simulink model "Csm_HighLvlArchitecture"  (R2017b)
settings: Solver=VariableStepAuto  StartTime=0.0  StopTime=10.0  RelTol=1e-3
undefined symbols (not defined in the file): accEgoVeh, Acceleration, apsEgoVeh, bpEgoVeh, Coasting, Control, CurrentDrivingLane, Curvature, CutIn, CutOut, Decelleration, distEgo2TS, distPredVeh, EgoVeh_State, EgoVehicle, GRG, Idle, ITS, Localization, Management, MATLAB, Mobileye, Obstacles, Obstacles_State, Perception, posEgoVeh, posGear, posTrafficSignal, PrecedingVehicle, Prediction, Python, Regen, Run, Slope, spdEgoVeh, spdMot, spdPredVeh, SpeedLimit, SRG, Stop, Topography, Topography_State, trqMot, Type, user_define_author, user_define_category, user_define_platform, Visual_C, yawEgoVeh
libraries: DX_Lib x1
(part 1 of 2)
settings Model: Creator=Haksu  LastModifiedBy=Haksu

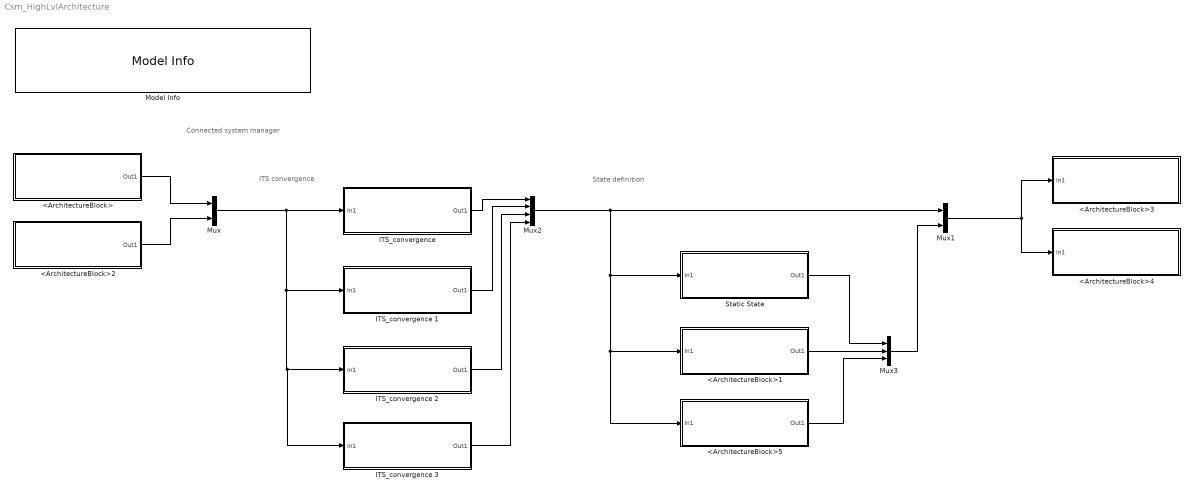
== system Csm_HighLvlArchitecture ==
  note: State definition
  note: ITS convergence
  note: Connected system manager
  <ArchitectureBlock> : Subsystem  mask{AlgorithmFullName=Localization, pop_author=__UserDef, editvalue_a=user_define_author, pop_platform=Visual_C, editvalue_p=user_define_platform, pop_category=__UserDef, editvalue_c=user_define_category, author_val=SRG, platform_val=Visual_C, algorithm_val=ITS}
      mask prompts: pop_author "Author"; editvalue_a "UserDefine"; pop_platform "Platform"; editvalue_p "UserDefine"; pop_category "Category"; editvalue_c "UserDefine"; author_val "Buff_author"; platform_val "Buff_Platform"; algorithm_val "Buff_Category"
      mask TypeOptions pop_author: Kyunghan | Haksu | Kyuhwan | Gyubin | Seungeon | __UserDef
      mask Callback pop_author:
      | % Get the mask parameter values. This is a cell
      | %   array of character vectors.
      | authorStr = get_param(gcb,'pop_author');
      | % The pop-up menu is the first mask parameter.
      | %   Check the value selected in the pop-up
      | if strcmp(authorStr(1),'_'),
      |     % Set the visibility of both parameters on when
      |     %   User-defined is selected in the pop-up.
      |     set_param(gcb,'editvalue_a','user_define_author');
      |     set_param(gcb,'MaskVisibilities',{'on';'on';'on';'on';'off';'on';'off';'off';'off';'off'}),
      |     % Get all Tab Names returned in cell array
      | 
      |     % Get visibility of all parameters
      | %     editvalStr = get_param(gcb,'editvalue')
      | %     set_param(gcb,'author_val',editvalStr)
      | else
      | 
      |     % Turn off the visibility of the Value field
      |     %   when User-defined is not selected.
      | 
      |     set_param(gcb,'MaskVisibilities',{'on';'on';'off';'on';'off';'on';'off';'off';'off';'off'}),
      |     % Set the character vector in the Values field equal to the
      |     % character vector selected in the Gain pop-up menu.
      | 
      |     %maskStr{2}=maskStr{1};
      | %     set_param(gcb,'author_val',authorStr);
      | end
      mask TypeOptions pop_platform: MATLAB | Python | Visual_C | __UserDef
      mask Callback pop_platform:
      | % Get the mask parameter values. This is a cell
      | %   array of character vectors.
      | platformSet = get_param(gcb,'pop_platform');
      | % The pop-up menu is the first mask parameter.
      | %   Check the value selected in the pop-up
      | if strcmp(platformSet(1),'_'),
      |     % Set the visibility of both parameters on when
      |     %   User-defined is selected in the pop-up.
      |     set_param(gcb,'editvalue_p','user_define_platform')
      |     set_param(gcb,'MaskVisibilities',{'on';'on';'off';'on';'on';'on';'off';'off';'off';'off'}),
      |     % Get all Tab Names returned in cell array
      | 
      |     % Get visibility of all parameters
      | %     editvalStr = get_param(gcb,'editvalue')
      | %     set_param(gcb,'platform_val',editvalStr)
      | else
      | 
      |     % Turn off the visibility of the Value field
      |     %   when User-defined is not selected.
      | 
      |     set_param(gcb,'MaskVisibilities',{'on';'on';'off';'on';'off';'on';'off';'off';'off';'off'}),
      |     % Set the character vector in the Values field equal to the
      |     % character vector selected in the Gain pop-up menu.
      | 
      |     %maskStr{2}=maskStr{1};
      | %     set_param(gcb,'platform_val',platformSet);
      | end
      mask TypeOptions pop_category: Management | Prediction | Control | __UserDef
      mask Callback pop_category:
      | % Get the mask parameter values. This is a cell
      | %   array of character vectors.
      | categoryset = get_param(gcb,'pop_category');
      | % The pop-up menu is the first mask parameter.
      | %   Check the value selected in the pop-up
      | if strcmp(categoryset(1),'_'),
      |     % Set the visibility of both parameters on when
      |     %   User-defined is selected in the pop-up.
      |     set_param(gcb,'editvalue_c','user_define_category')
      |     set_param(gcb,'MaskVisibilities',{'on';'on';'off';'on';'off';'on';'on';'off';'off';'off'}),
      |     % Get all Tab Names returned in cell array
      | else
      |     % Turn off the visibility of the Value field
      |     %   when User-defined is not selected.
      |     set_param(gcb,'MaskVisibilities',{'on';'on';'off';'on';'off';'on';'off';'off';'off';'off'}),
      |     % Set the character vector in the Values field equal to the
      |     % character vector selected in the Gain pop-up menu.
      |     %maskStr{2}=maskStr{1};
      | end
      mask DialogControl DescGroupVar Prompt: Description
      mask DialogControl DescTextVar Prompt: %<AlgorithmFullName>
      mask DialogControl ParamDesc Prompt: Description
      mask DialogControl Text1 Prompt: Author: %<author_val>
      mask DialogControl Text2 Prompt: Platform: %<platform_val>
      mask DialogControl Text3 Prompt: Algorithm: %<algorithm_val>
      mask DialogControl ParameterGroupVar Prompt: SetParam
      mask DialogControl Control5 Prompt: Set
      mask DialogControl Control5 Callback:
      | authorset = get_param(gcb,'pop_author');
      | platformset = get_param(gcb,'pop_platform');
      | categoryset = get_param(gcb,'pop_category');
      | % The pop-up menu is the first mask parameter.
      | %   Check the value selected in the pop-up
      | if strcmp(authorset(1),'_'),
      |     editvalStr = get_param(gcb,'editvalue_a');
      |     set_param(gcb,'author_val',editvalStr);
      | else
      |     set_param(gcb,'author_val',authorset);
      | end
      | 
      | if strcmp(platformset(1),'_'),
      |     editvalStr = get_param(gcb,'editvalue_p');
      |     set_param(gcb,'platform_val',editvalStr);
      | else
      |     set_param(gcb,'platform_val',platformset);
      | end
      | 
      | if strcmp(categoryset(1),'_'),
      |     editvalStr = get_param(gcb,'editvalue_c');
      |     set_param(gcb,'algorithm_val',editvalStr);
      | else
      |     set_param(gcb,'algorithm_val',categoryset);
      | end
      mask Display:
      | val_dis_author = get_param(gcb,'author_val');
      | val_dis_plat = get_param(gcb,'platform_val');
      | val_dis_cat = get_param(gcb,'algorithm_val');
      | val_dis_desc = get_param(gcb,'AlgorithmFullName');
      | 
      | colorstr = 'black';
      | switch(val_dis_cat)
      |     case 'Management'
      |         colorstr = 'lightblue';
      |     case 'Prediction'
      |         colorstr = 'blue';
      |     case 'Control'
      |         colorstr = 'green';
      |     otherwise
      |         colorstr = 'yellow';
      | end
      | 
      | % if val_dis_cat == 'Management'
      | %     colorstr = 'lightblue';
      | % end
      | % if val_dis_cat == 'Prediction'
      | %     colorstr = 'blue';
      | % end
      | 
      | % if val_dis_cat == 'Control'
      | %     colorstr = 'blue';
      | % end
      | % if val_dis_cat == 'Control'
      | %     colorstr = 'green';
      | % end
      | 
      | color(colorstr);
      | text(0.5,0.9,val_dis_desc,'horizontalAlignment', 'center', 'VerticalAlignment','Top');
      | color('black');
      | fprintf('\nAuthor: %s\nPlatform: %s\nCategory: %s',val_dis_author,val_dis_plat,val_dis_cat);
  <ArchitectureBlock>1 : Subsystem  mask{AlgorithmFullName=Obstacles_State, pop_author=__UserDef, editvalue_a=user_define_author, pop_platform=Python, editvalue_p=user_define_platform, pop_category=Management, editvalue_c=user_define_category, author_val=user_define_author, platform_val=Python, algorithm_val=Management}
      mask prompts: pop_author "Author"; editvalue_a "UserDefine"; pop_platform "Platform"; editvalue_p "UserDefine"; pop_category "Category"; editvalue_c "UserDefine"; author_val "Buff_author"; platform_val "Buff_Platform"; algorithm_val "Buff_Category"
      mask TypeOptions pop_author: Kyunghan | Haksu | Kyuhwan | Gyubin | Seungeon | __UserDef
      mask Callback pop_author:
      | % Get the mask parameter values. This is a cell
      | %   array of character vectors.
      | authorStr = get_param(gcb,'pop_author');
      | % The pop-up menu is the first mask parameter.
      | %   Check the value selected in the pop-up
      | if strcmp(authorStr(1),'_'),
      |     % Set the visibility of both parameters on when
      |     %   User-defined is selected in the pop-up.
      |     set_param(gcb,'editvalue_a','user_define_author');
      |     set_param(gcb,'MaskVisibilities',{'on';'on';'on';'on';'off';'on';'off';'off';'off';'off'}),
      |     % Get all Tab Names returned in cell array
      | 
      |     % Get visibility of all parameters
      | %     editvalStr = get_param(gcb,'editvalue')
      | %     set_param(gcb,'author_val',editvalStr)
      | else
      | 
      |     % Turn off the visibility of the Value field
      |     %   when User-defined is not selected.
      | 
      |     set_param(gcb,'MaskVisibilities',{'on';'on';'off';'on';'off';'on';'off';'off';'off';'off'}),
      |     % Set the character vector in the Values field equal to the
      |     % character vector selected in the Gain pop-up menu.
      | 
      |     %maskStr{2}=maskStr{1};
      | %     set_param(gcb,'author_val',authorStr);
      | end
      mask TypeOptions pop_platform: MATLAB | Python | Visual_C | __UserDef
      mask Callback pop_platform:
      | % Get the mask parameter values. This is a cell
      | %   array of character vectors.
      | platformSet = get_param(gcb,'pop_platform');
      | % The pop-up menu is the first mask parameter.
      | %   Check the value selected in the pop-up
      | if strcmp(platformSet(1),'_'),
      |     % Set the visibility of both parameters on when
      |     %   User-defined is selected in the pop-up.
      |     set_param(gcb,'editvalue_p','user_define_platform')
      |     set_param(gcb,'MaskVisibilities',{'on';'on';'off';'on';'on';'on';'off';'off';'off';'off'}),
      |     % Get all Tab Names returned in cell array
      | 
      |     % Get visibility of all parameters
      | %     editvalStr = get_param(gcb,'editvalue')
      | %     set_param(gcb,'platform_val',editvalStr)
      | else
      | 
      |     % Turn off the visibility of the Value field
      |     %   when User-defined is not selected.
      | 
      |     set_param(gcb,'MaskVisibilities',{'on';'on';'off';'on';'off';'on';'off';'off';'off';'off'}),
      |     % Set the character vector in the Values field equal to the
      |     % character vector selected in the Gain pop-up menu.
      | 
      |     %maskStr{2}=maskStr{1};
      | %     set_param(gcb,'platform_val',platformSet);
      | end
      mask TypeOptions pop_category: Management | Prediction | Control | __UserDef
      mask Callback pop_category:
      | % Get the mask parameter values. This is a cell
      | %   array of character vectors.
      | categoryset = get_param(gcb,'pop_category');
      | % The pop-up menu is the first mask parameter.
      | %   Check the value selected in the pop-up
      | if strcmp(categoryset(1),'_'),
      |     % Set the visibility of both parameters on when
      |     %   User-defined is selected in the pop-up.
      |     set_param(gcb,'editvalue_c','user_define_category')
      |     set_param(gcb,'MaskVisibilities',{'on';'on';'off';'on';'off';'on';'on';'off';'off';'off'}),
      |     % Get all Tab Names returned in cell array
      | else
      |     % Turn off the visibility of the Value field
      |     %   when User-defined is not selected.
      |     set_param(gcb,'MaskVisibilities',{'on';'on';'off';'on';'off';'on';'off';'off';'off';'off'}),
      |     % Set the character vector in the Values field equal to the
      |     % character vector selected in the Gain pop-up menu.
      |     %maskStr{2}=maskStr{1};
      | end
      mask DialogControl DescGroupVar Prompt: Description
      mask DialogControl DescTextVar Prompt: %<AlgorithmFullName>
      mask DialogControl ParamDesc Prompt: Description
      mask DialogControl Text1 Prompt: Author: %<author_val>
      mask DialogControl Text2 Prompt: Platform: %<platform_val>
      mask DialogControl Text3 Prompt: Algorithm: %<algorithm_val>
      mask DialogControl ParameterGroupVar Prompt: SetParam
      mask DialogControl Control5 Prompt: Set
      mask DialogControl Control5 Callback:
      | authorset = get_param(gcb,'pop_author');
      | platformset = get_param(gcb,'pop_platform');
      | categoryset = get_param(gcb,'pop_category');
      | % The pop-up menu is the first mask parameter.
      | %   Check the value selected in the pop-up
      | if strcmp(authorset(1),'_'),
      |     editvalStr = get_param(gcb,'editvalue_a');
      |     set_param(gcb,'author_val',editvalStr);
      | else
      |     set_param(gcb,'author_val',authorset);
      | end
      | 
      | if strcmp(platformset(1),'_'),
      |     editvalStr = get_param(gcb,'editvalue_p');
      |     set_param(gcb,'platform_val',editvalStr);
      | else
      |     set_param(gcb,'platform_val',platformset);
      | end
      | 
      | if strcmp(categoryset(1),'_'),
      |     editvalStr = get_param(gcb,'editvalue_c');
      |     set_param(gcb,'algorithm_val',editvalStr);
      | else
      |     set_param(gcb,'algorithm_val',categoryset);
      | end
      mask Display:
      | val_dis_author = get_param(gcb,'author_val');
      | val_dis_plat = get_param(gcb,'platform_val');
      | val_dis_cat = get_param(gcb,'algorithm_val');
      | val_dis_desc = get_param(gcb,'AlgorithmFullName');
      | 
      | colorstr = 'black';
      | switch(val_dis_cat)
      |     case 'Management'
      |         colorstr = 'lightblue';
      |     case 'Prediction'
      |         colorstr = 'blue';
      |     case 'Control'
      |         colorstr = 'green';
      |     otherwise
      |         colorstr = 'yellow';
      | end
      | 
      | % if val_dis_cat == 'Management'
      | %     colorstr = 'lightblue';
      | % end
      | % if val_dis_cat == 'Prediction'
      | %     colorstr = 'blue';
      | % end
      | 
      | % if val_dis_cat == 'Control'
      | %     colorstr = 'blue';
      | % end
      | % if val_dis_cat == 'Control'
      | %     colorstr = 'green';
      | % end
      | 
      | color(colorstr);
      | text(0.5,0.9,val_dis_desc,'horizontalAlignment', 'center', 'VerticalAlignment','Top');
      | color('black');
      | fprintf('\nAuthor: %s\nPlatform: %s\nCategory: %s',val_dis_author,val_dis_plat,val_dis_cat);
  <ArchitectureBlock>2 : Subsystem  mask{AlgorithmFullName=Perception, pop_author=__UserDef, editvalue_a=user_define_author, pop_platform=Visual_C, editvalue_p=user_define_platform, pop_category=__UserDef, editvalue_c=user_define_category, author_val=SRG, platform_val=Visual_C, algorithm_val=ITS}
      mask prompts: pop_author "Author"; editvalue_a "UserDefine"; pop_platform "Platform"; editvalue_p "UserDefine"; pop_category "Category"; editvalue_c "UserDefine"; author_val "Buff_author"; platform_val "Buff_Platform"; algorithm_val "Buff_Category"
      mask TypeOptions pop_author: Kyunghan | Haksu | Kyuhwan | Gyubin | Seungeon | __UserDef
      mask Callback pop_author:
      | % Get the mask parameter values. This is a cell
      | %   array of character vectors.
      | authorStr = get_param(gcb,'pop_author');
      | % The pop-up menu is the first mask parameter.
      | %   Check the value selected in the pop-up
      | if strcmp(authorStr(1),'_'),
      |     % Set the visibility of both parameters on when
      |     %   User-defined is selected in the pop-up.
      |     set_param(gcb,'editvalue_a','user_define_author');
      |     set_param(gcb,'MaskVisibilities',{'on';'on';'on';'on';'off';'on';'off';'off';'off';'off'}),
      |     % Get all Tab Names returned in cell array
      | 
      |     % Get visibility of all parameters
      | %     editvalStr = get_param(gcb,'editvalue')
      | %     set_param(gcb,'author_val',editvalStr)
      | else
      | 
      |     % Turn off the visibility of the Value field
      |     %   when User-defined is not selected.
      | 
      |     set_param(gcb,'MaskVisibilities',{'on';'on';'off';'on';'off';'on';'off';'off';'off';'off'}),
      |     % Set the character vector in the Values field equal to the
      |     % character vector selected in the Gain pop-up menu.
      | 
      |     %maskStr{2}=maskStr{1};
      | %     set_param(gcb,'author_val',authorStr);
      | end
      mask TypeOptions pop_platform: MATLAB | Python | Visual_C | __UserDef
      mask Callback pop_platform:
      | % Get the mask parameter values. This is a cell
      | %   array of character vectors.
      | platformSet = get_param(gcb,'pop_platform');
      | % The pop-up menu is the first mask parameter.
      | %   Check the value selected in the pop-up
      | if strcmp(platformSet(1),'_'),
      |     % Set the visibility of both parameters on when
      |     %   User-defined is selected in the pop-up.
      |     set_param(gcb,'editvalue_p','user_define_platform')
      |     set_param(gcb,'MaskVisibilities',{'on';'on';'off';'on';'on';'on';'off';'off';'off';'off'}),
      |     % Get all Tab Names returned in cell array
      | 
      |     % Get visibility of all parameters
      | %     editvalStr = get_param(gcb,'editvalue')
      | %     set_param(gcb,'platform_val',editvalStr)
      | else
      | 
      |     % Turn off the visibility of the Value field
      |     %   when User-defined is not selected.
      | 
      |     set_param(gcb,'MaskVisibilities',{'on';'on';'off';'on';'off';'on';'off';'off';'off';'off'}),
      |     % Set the character vector in the Values field equal to the
      |     % character vector selected in the Gain pop-up menu.
      | 
      |     %maskStr{2}=maskStr{1};
      | %     set_param(gcb,'platform_val',platformSet);
      | end
      mask TypeOptions pop_category: Management | Prediction | Control | __UserDef
      mask Callback pop_category:
      | % Get the mask parameter values. This is a cell
      | %   array of character vectors.
      | categoryset = get_param(gcb,'pop_category');
      | % The pop-up menu is the first mask parameter.
      | %   Check the value selected in the pop-up
      | if strcmp(categoryset(1),'_'),
      |     % Set the visibility of both parameters on when
      |     %   User-defined is selected in the pop-up.
      |     set_param(gcb,'editvalue_c','user_define_category')
      |     set_param(gcb,'MaskVisibilities',{'on';'on';'off';'on';'off';'on';'on';'off';'off';'off'}),
      |     % Get all Tab Names returned in cell array
      | else
      |     % Turn off the visibility of the Value field
      |     %   when User-defined is not selected.
      |     set_param(gcb,'MaskVisibilities',{'on';'on';'off';'on';'off';'on';'off';'off';'off';'off'}),
      |     % Set the character vector in the Values field equal to the
      |     % character vector selected in the Gain pop-up menu.
      |     %maskStr{2}=maskStr{1};
      | end
      mask DialogControl DescGroupVar Prompt: Description
      mask DialogControl DescTextVar Prompt: %<AlgorithmFullName>
      mask DialogControl ParamDesc Prompt: Description
      mask DialogControl Text1 Prompt: Author: %<author_val>
      mask DialogControl Text2 Prompt: Platform: %<platform_val>
      mask DialogControl Text3 Prompt: Algorithm: %<algorithm_val>
      mask DialogControl ParameterGroupVar Prompt: SetParam
      mask DialogControl Control5 Prompt: Set
      mask DialogControl Control5 Callback:
      | authorset = get_param(gcb,'pop_author');
      | platformset = get_param(gcb,'pop_platform');
      | categoryset = get_param(gcb,'pop_category');
      | % The pop-up menu is the first mask parameter.
      | %   Check the value selected in the pop-up
      | if strcmp(authorset(1),'_'),
      |     editvalStr = get_param(gcb,'editvalue_a');
      |     set_param(gcb,'author_val',editvalStr);
      | else
      |     set_param(gcb,'author_val',authorset);
      | end
      | 
      | if strcmp(platformset(1),'_'),
      |     editvalStr = get_param(gcb,'editvalue_p');
      |     set_param(gcb,'platform_val',editvalStr);
      | else
      |     set_param(gcb,'platform_val',platformset);
      | end
      | 
      | if strcmp(categoryset(1),'_'),
      |     editvalStr = get_param(gcb,'editvalue_c');
      |     set_param(gcb,'algorithm_val',editvalStr);
      | else
      |     set_param(gcb,'algorithm_val',categoryset);
      | end
      mask Display:
      | val_dis_author = get_param(gcb,'author_val');
      | val_dis_plat = get_param(gcb,'platform_val');
      | val_dis_cat = get_param(gcb,'algorithm_val');
      | val_dis_desc = get_param(gcb,'AlgorithmFullName');
      | 
      | colorstr = 'black';
      | switch(val_dis_cat)
      |     case 'Management'
      |         colorstr = 'lightblue';
      |     case 'Prediction'
      |         colorstr = 'blue';
      |     case 'Control'
      |         colorstr = 'green';
      |     otherwise
      |         colorstr = 'yellow';
      | end
      | 
      | % if val_dis_cat == 'Management'
      | %     colorstr = 'lightblue';
      | % end
      | % if val_dis_cat == 'Prediction'
      | %     colorstr = 'blue';
      | % end
      | 
      | % if val_dis_cat == 'Control'
      | %     colorstr = 'blue';
      | % end
      | % if val_dis_cat == 'Control'
      | %     colorstr = 'green';
      | % end
      | 
      | color(colorstr);
      | text(0.5,0.9,val_dis_desc,'horizontalAlignment', 'center', 'VerticalAlignment','Top');
      | color('black');
      | fprintf('\nAuthor: %s\nPlatform: %s\nCategory: %s',val_dis_author,val_dis_plat,val_dis_cat);
  <ArchitectureBlock>3 : Subsystem  mask{AlgorithmFullName=Prediction, pop_author=__UserDef, editvalue_a=user_define_author, pop_platform=MATLAB, editvalue_p=user_define_platform, pop_category=Prediction, editvalue_c=user_define_category, author_val=GRG, platform_val=MATLAB, algorithm_val=Prediction}
      mask prompts: pop_author "Author"; editvalue_a "UserDefine"; pop_platform "Platform"; editvalue_p "UserDefine"; pop_category "Category"; editvalue_c "UserDefine"; author_val "Buff_author"; platform_val "Buff_Platform"; algorithm_val "Buff_Category"
      mask TypeOptions pop_author: Kyunghan | Haksu | Kyuhwan | Gyubin | Seungeon | __UserDef
      mask Callback pop_author:
      | % Get the mask parameter values. This is a cell
      | %   array of character vectors.
      | authorStr = get_param(gcb,'pop_author');
      | % The pop-up menu is the first mask parameter.
      | %   Check the value selected in the pop-up
      | if strcmp(authorStr(1),'_'),
      |     % Set the visibility of both parameters on when
      |     %   User-defined is selected in the pop-up.
      |     set_param(gcb,'editvalue_a','user_define_author');
      |     set_param(gcb,'MaskVisibilities',{'on';'on';'on';'on';'off';'on';'off';'off';'off';'off'}),
      |     % Get all Tab Names returned in cell array
      | 
      |     % Get visibility of all parameters
      | %     editvalStr = get_param(gcb,'editvalue')
      | %     set_param(gcb,'author_val',editvalStr)
      | else
      | 
      |     % Turn off the visibility of the Value field
      |     %   when User-defined is not selected.
      | 
      |     set_param(gcb,'MaskVisibilities',{'on';'on';'off';'on';'off';'on';'off';'off';'off';'off'}),
      |     % Set the character vector in the Values field equal to the
      |     % character vector selected in the Gain pop-up menu.
      | 
      |     %maskStr{2}=maskStr{1};
      | %     set_param(gcb,'author_val',authorStr);
      | end
      mask TypeOptions pop_platform: MATLAB | Python | Visual_C | __UserDef
      mask Callback pop_platform:
      | % Get the mask parameter values. This is a cell
      | %   array of character vectors.
      | platformSet = get_param(gcb,'pop_platform');
      | % The pop-up menu is the first mask parameter.
      | %   Check the value selected in the pop-up
      | if strcmp(platformSet(1),'_'),
      |     % Set the visibility of both parameters on when
      |     %   User-defined is selected in the pop-up.
      |     set_param(gcb,'editvalue_p','user_define_platform')
      |     set_param(gcb,'MaskVisibilities',{'on';'on';'off';'on';'on';'on';'off';'off';'off';'off'}),
      |     % Get all Tab Names returned in cell array
      | 
      |     % Get visibility of all parameters
      | %     editvalStr = get_param(gcb,'editvalue')
      | %     set_param(gcb,'platform_val',editvalStr)
      | else
      | 
      |     % Turn off the visibility of the Value field
      |     %   when User-defined is not selected.
      | 
      |     set_param(gcb,'MaskVisibilities',{'on';'on';'off';'on';'off';'on';'off';'off';'off';'off'}),
      |     % Set the character vector in the Values field equal to the
      |     % character vector selected in the Gain pop-up menu.
      | 
      |     %maskStr{2}=maskStr{1};
      | %     set_param(gcb,'platform_val',platformSet);
      | end
      mask TypeOptions pop_category: Management | Prediction | Control | __UserDef
      mask Callback pop_category:
      | % Get the mask parameter values. This is a cell
      | %   array of character vectors.
      | categoryset = get_param(gcb,'pop_category');
      | % The pop-up menu is the first mask parameter.
      | %   Check the value selected in the pop-up
      | if strcmp(categoryset(1),'_'),
      |     % Set the visibility of both parameters on when
      |     %   User-defined is selected in the pop-up.
      |     set_param(gcb,'editvalue_c','user_define_category')
      |     set_param(gcb,'MaskVisibilities',{'on';'on';'off';'on';'off';'on';'on';'off';'off';'off'}),
      |     % Get all Tab Names returned in cell array
      | else
      |     % Turn off the visibility of the Value field
      |     %   when User-defined is not selected.
      |     set_param(gcb,'MaskVisibilities',{'on';'on';'off';'on';'off';'on';'off';'off';'off';'off'}),
      |     % Set the character vector in the Values field equal to the
      |     % character vector selected in the Gain pop-up menu.
      |     %maskStr{2}=maskStr{1};
      | end
      mask DialogControl DescGroupVar Prompt: Description
      mask DialogControl DescTextVar Prompt: %<AlgorithmFullName>
      mask DialogControl ParamDesc Prompt: Description
      mask DialogControl Text1 Prompt: Author: %<author_val>
      mask DialogControl Text2 Prompt: Platform: %<platform_val>
      mask DialogControl Text3 Prompt: Algorithm: %<algorithm_val>
      mask DialogControl ParameterGroupVar Prompt: SetParam
      mask DialogControl Control5 Prompt: Set
      mask DialogControl Control5 Callback:
      | authorset = get_param(gcb,'pop_author');
      | platformset = get_param(gcb,'pop_platform');
      | categoryset = get_param(gcb,'pop_category');
      | % The pop-up menu is the first mask parameter.
      | %   Check the value selected in the pop-up
      | if strcmp(authorset(1),'_'),
      |     editvalStr = get_param(gcb,'editvalue_a');
      |     set_param(gcb,'author_val',editvalStr);
      | else
      |     set_param(gcb,'author_val',authorset);
      | end
      | 
      | if strcmp(platformset(1),'_'),
      |     editvalStr = get_param(gcb,'editvalue_p');
      |     set_param(gcb,'platform_val',editvalStr);
      | else
      |     set_param(gcb,'platform_val',platformset);
      | end
      | 
      | if strcmp(categoryset(1),'_'),
      |     editvalStr = get_param(gcb,'editvalue_c');
      |     set_param(gcb,'algorithm_val',editvalStr);
      | else
      |     set_param(gcb,'algorithm_val',categoryset);
      | end
      mask Display:
      | val_dis_author = get_param(gcb,'author_val');
      | val_dis_plat = get_param(gcb,'platform_val');
      | val_dis_cat = get_param(gcb,'algorithm_val');
      | val_dis_desc = get_param(gcb,'AlgorithmFullName');
      | 
      | colorstr = 'black';
      | switch(val_dis_cat)
      |     case 'Management'
      |         colorstr = 'lightblue';
      |     case 'Prediction'
      |         colorstr = 'blue';
      |     case 'Control'
      |         colorstr = 'green';
      |     otherwise
      |         colorstr = 'yellow';
      | end
      | 
      | % if val_dis_cat == 'Management'
      | %     colorstr = 'lightblue';
      | % end
      | % if val_dis_cat == 'Prediction'
      | %     colorstr = 'blue';
      | % end
      | 
      | % if val_dis_cat == 'Control'
      | %     colorstr = 'blue';
      | % end
      | % if val_dis_cat == 'Control'
      | %     colorstr = 'green';
      | % end
      | 
      | color(colorstr);
      | text(0.5,0.9,val_dis_desc,'horizontalAlignment', 'center', 'VerticalAlignment','Top');
      | color('black');
      | fprintf('\nAuthor: %s\nPlatform: %s\nCategory: %s',val_dis_author,val_dis_plat,val_dis_cat);
  <ArchitectureBlock>4 : Subsystem  mask{AlgorithmFullName=Control, pop_author=__UserDef, editvalue_a=GRG, pop_platform=MATLAB, editvalue_p=user_define_platform, pop_category=Control, editvalue_c=user_define_category, author_val=GRG, platform_val=MATLAB, algorithm_val=Control}
      mask prompts: pop_author "Author"; editvalue_a "UserDefine"; pop_platform "Platform"; editvalue_p "UserDefine"; pop_category "Category"; editvalue_c "UserDefine"; author_val "Buff_author"; platform_val "Buff_Platform"; algorithm_val "Buff_Category"
      mask TypeOptions pop_author: Kyunghan | Haksu | Kyuhwan | Gyubin | Seungeon | __UserDef
      mask Callback pop_author:
      | % Get the mask parameter values. This is a cell
      | %   array of character vectors.
      | authorStr = get_param(gcb,'pop_author');
      | % The pop-up menu is the first mask parameter.
      | %   Check the value selected in the pop-up
      | if strcmp(authorStr(1),'_'),
      |     % Set the visibility of both parameters on when
      |     %   User-defined is selected in the pop-up.
      |     set_param(gcb,'editvalue_a','user_define_author');
      |     set_param(gcb,'MaskVisibilities',{'on';'on';'on';'on';'off';'on';'off';'off';'off';'off'}),
      |     % Get all Tab Names returned in cell array
      | 
      |     % Get visibility of all parameters
      | %     editvalStr = get_param(gcb,'editvalue')
      | %     set_param(gcb,'author_val',editvalStr)
      | else
      | 
      |     % Turn off the visibility of the Value field
      |     %   when User-defined is not selected.
      | 
      |     set_param(gcb,'MaskVisibilities',{'on';'on';'off';'on';'off';'on';'off';'off';'off';'off'}),
      |     % Set the character vector in the Values field equal to the
      |     % character vector selected in the Gain pop-up menu.
      | 
      |     %maskStr{2}=maskStr{1};
      | %     set_param(gcb,'author_val',authorStr);
      | end
      mask TypeOptions pop_platform: MATLAB | Python | Visual_C | __UserDef
      mask Callback pop_platform:
      | % Get the mask parameter values. This is a cell
      | %   array of character vectors.
      | platformSet = get_param(gcb,'pop_platform');
      | % The pop-up menu is the first mask parameter.
      | %   Check the value selected in the pop-up
      | if strcmp(platformSet(1),'_'),
      |     % Set the visibility of both parameters on when
      |     %   User-defined is selected in the pop-up.
      |     set_param(gcb,'editvalue_p','user_define_platform')
      |     set_param(gcb,'MaskVisibilities',{'on';'on';'off';'on';'on';'on';'off';'off';'off';'off'}),
      |     % Get all Tab Names returned in cell array
      | 
      |     % Get visibility of all parameters
      | %     editvalStr = get_param(gcb,'editvalue')
      | %     set_param(gcb,'platform_val',editvalStr)
      | else
      | 
      |     % Turn off the visibility of the Value field
      |     %   when User-defined is not selected.
      | 
      |     set_param(gcb,'MaskVisibilities',{'on';'on';'off';'on';'off';'on';'off';'off';'off';'off'}),
      |     % Set the character vector in the Values field equal to the
      |     % character vector selected in the Gain pop-up menu.
      | 
      |     %maskStr{2}=maskStr{1};
      | %     set_param(gcb,'platform_val',platformSet);
      | end
      mask TypeOptions pop_category: Management | Prediction | Control | __UserDef
      mask Callback pop_category:
      | % Get the mask parameter values. This is a cell
      | %   array of character vectors.
      | categoryset = get_param(gcb,'pop_category');
      | % The pop-up menu is the first mask parameter.
      | %   Check the value selected in the pop-up
      | if strcmp(categoryset(1),'_'),
      |     % Set the visibility of both parameters on when
      |     %   User-defined is selected in the pop-up.
      |     set_param(gcb,'editvalue_c','user_define_category')
      |     set_param(gcb,'MaskVisibilities',{'on';'on';'off';'on';'off';'on';'on';'off';'off';'off'}),
      |     % Get all Tab Names returned in cell array
      | else
      |     % Turn off the visibility of the Value field
      |     %   when User-defined is not selected.
      |     set_param(gcb,'MaskVisibilities',{'on';'on';'off';'on';'off';'on';'off';'off';'off';'off'}),
      |     % Set the character vector in the Values field equal to the
      |     % character vector selected in the Gain pop-up menu.
      |     %maskStr{2}=maskStr{1};
      | end
      mask DialogControl DescGroupVar Prompt: Description
      mask DialogControl DescTextVar Prompt: %<AlgorithmFullName>
      mask DialogControl ParamDesc Prompt: Description
      mask DialogControl Text1 Prompt: Author: %<author_val>
      mask DialogControl Text2 Prompt: Platform: %<platform_val>
      mask DialogControl Text3 Prompt: Algorithm: %<algorithm_val>
      mask DialogControl ParameterGroupVar Prompt: SetParam
      mask DialogControl Control5 Prompt: Set
      mask DialogControl Control5 Callback:
      | authorset = get_param(gcb,'pop_author');
      | platformset = get_param(gcb,'pop_platform');
      | categoryset = get_param(gcb,'pop_category');
      | % The pop-up menu is the first mask parameter.
      | %   Check the value selected in the pop-up
      | if strcmp(authorset(1),'_'),
      |     editvalStr = get_param(gcb,'editvalue_a');
      |     set_param(gcb,'author_val',editvalStr);
      | else
      |     set_param(gcb,'author_val',authorset);
      | end
      | 
      | if strcmp(platformset(1),'_'),
      |     editvalStr = get_param(gcb,'editvalue_p');
      |     set_param(gcb,'platform_val',editvalStr);
      | else
      |     set_param(gcb,'platform_val',platformset);
      | end
      | 
      | if strcmp(categoryset(1),'_'),
      |     editvalStr = get_param(gcb,'editvalue_c');
      |     set_param(gcb,'algorithm_val',editvalStr);
      | else
      |     set_param(gcb,'algorithm_val',categoryset);
      | end
      mask Display:
      | val_dis_author = get_param(gcb,'author_val');
      | val_dis_plat = get_param(gcb,'platform_val');
      | val_dis_cat = get_param(gcb,'algorithm_val');
      | val_dis_desc = get_param(gcb,'AlgorithmFullName');
      | 
      | colorstr = 'black';
      | switch(val_dis_cat)
      |     case 'Management'
      |         colorstr = 'lightblue';
      |     case 'Prediction'
      |         colorstr = 'blue';
      |     case 'Control'
      |         colorstr = 'green';
      |     otherwise
      |         colorstr = 'yellow';
      | end
      | 
      | % if val_dis_cat == 'Management'
      | %     colorstr = 'lightblue';
      | % end
      | % if val_dis_cat == 'Prediction'
      | %     colorstr = 'blue';
      | % end
      | 
      | % if val_dis_cat == 'Control'
      | %     colorstr = 'blue';
      | % end
      | % if val_dis_cat == 'Control'
      | %     colorstr = 'green';
      | % end
      | 
      | color(colorstr);
      | text(0.5,0.9,val_dis_desc,'horizontalAlignment', 'center', 'VerticalAlignment','Top');
      | color('black');
      | fprintf('\nAuthor: %s\nPlatform: %s\nCategory: %s',val_dis_author,val_dis_plat,val_dis_cat);
  <ArchitectureBlock>5 : Subsystem  mask{AlgorithmFullName=Topography_State, pop_author=__UserDef, editvalue_a=user_define_author, pop_platform=Python, editvalue_p=user_define_platform, pop_category=Management, editvalue_c=user_define_category, author_val=user_define_author, platform_val=Python, algorithm_val=Management}
      mask prompts: pop_author "Author"; editvalue_a "UserDefine"; pop_platform "Platform"; editvalue_p "UserDefine"; pop_category "Category"; editvalue_c "UserDefine"; author_val "Buff_author"; platform_val "Buff_Platform"; algorithm_val "Buff_Category"
      mask TypeOptions pop_author: Kyunghan | Haksu | Kyuhwan | Gyubin | Seungeon | __UserDef
      mask Callback pop_author:
      | % Get the mask parameter values. This is a cell
      | %   array of character vectors.
      | authorStr = get_param(gcb,'pop_author');
      | % The pop-up menu is the first mask parameter.
      | %   Check the value selected in the pop-up
      | if strcmp(authorStr(1),'_'),
      |     % Set the visibility of both parameters on when
      |     %   User-defined is selected in the pop-up.
      |     set_param(gcb,'editvalue_a','user_define_author');
      |     set_param(gcb,'MaskVisibilities',{'on';'on';'on';'on';'off';'on';'off';'off';'off';'off'}),
      |     % Get all Tab Names returned in cell array
      | 
      |     % Get visibility of all parameters
      | %     editvalStr = get_param(gcb,'editvalue')
      | %     set_param(gcb,'author_val',editvalStr)
      | else
      | 
      |     % Turn off the visibility of the Value field
      |     %   when User-defined is not selected.
      | 
      |     set_param(gcb,'MaskVisibilities',{'on';'on';'off';'on';'off';'on';'off';'off';'off';'off'}),
      |     % Set the character vector in the Values field equal to the
      |     % character vector selected in the Gain pop-up menu.
      | 
      |     %maskStr{2}=maskStr{1};
      | %     set_param(gcb,'author_val',authorStr);
      | end
      mask TypeOptions pop_platform: MATLAB | Python | Visual_C | __UserDef
      mask Callback pop_platform:
      | % Get the mask parameter values. This is a cell
      | %   array of character vectors.
      | platformSet = get_param(gcb,'pop_platform');
      | % The pop-up menu is the first mask parameter.
      | %   Check the value selected in the pop-up
      | if strcmp(platformSet(1),'_'),
      |     % Set the visibility of both parameters on when
      |     %   User-defined is selected in the pop-up.
      |     set_param(gcb,'editvalue_p','user_define_platform')
      |     set_param(gcb,'MaskVisibilities',{'on';'on';'off';'on';'on';'on';'off';'off';'off';'off'}),
      |     % Get all Tab Names returned in cell array
      | 
      |     % Get visibility of all parameters
      | %     editvalStr = get_param(gcb,'editvalue')
      | %     set_param(gcb,'platform_val',editvalStr)
      | else
      | 
      |     % Turn off the visibility of the Value field
      |     %   when User-defined is not selected.
      | 
      |     set_param(gcb,'MaskVisibilities',{'on';'on';'off';'on';'off';'on';'off';'off';'off';'off'}),
      |     % Set the character vector in the Values field equal to the
      |     % character vector selected in the Gain pop-up menu.
      | 
      |     %maskStr{2}=maskStr{1};
      | %     set_param(gcb,'platform_val',platformSet);
      | end
      mask TypeOptions pop_category: Management | Prediction | Control | __UserDef
      mask Callback pop_category:
      | % Get the mask parameter values. This is a cell
      | %   array of character vectors.
      | categoryset = get_param(gcb,'pop_category');
      | % The pop-up menu is the first mask parameter.
      | %   Check the value selected in the pop-up
      | if strcmp(categoryset(1),'_'),
      |     % Set the visibility of both parameters on when
      |     %   User-defined is selected in the pop-up.
      |     set_param(gcb,'editvalue_c','user_define_category')
      |     set_param(gcb,'MaskVisibilities',{'on';'on';'off';'on';'off';'on';'on';'off';'off';'off'}),
      |     % Get all Tab Names returned in cell array
      | else
      |     % Turn off the visibility of the Value field
      |     %   when User-defined is not selected.
      |     set_param(gcb,'MaskVisibilities',{'on';'on';'off';'on';'off';'on';'off';'off';'off';'off'}),
      |     % Set the character vector in the Values field equal to the
      |     % character vector selected in the Gain pop-up menu.
      |     %maskStr{2}=maskStr{1};
      | end
      mask DialogControl DescGroupVar Prompt: Description
      mask DialogControl DescTextVar Prompt: %<AlgorithmFullName>
      mask DialogControl ParamDesc Prompt: Description
      mask DialogControl Text1 Prompt: Author: %<author_val>
      mask DialogControl Text2 Prompt: Platform: %<platform_val>
      mask DialogControl Text3 Prompt: Algorithm: %<algorithm_val>
      mask DialogControl ParameterGroupVar Prompt: SetParam
      mask DialogControl Control5 Prompt: Set
      mask DialogControl Control5 Callback:
      | authorset = get_param(gcb,'pop_author');
      | platformset = get_param(gcb,'pop_platform');
      | categoryset = get_param(gcb,'pop_category');
      | % The pop-up menu is the first mask parameter.
      | %   Check the value selected in the pop-up
      | if strcmp(authorset(1),'_'),
      |     editvalStr = get_param(gcb,'editvalue_a');
      |     set_param(gcb,'author_val',editvalStr);
      | else
      |     set_param(gcb,'author_val',authorset);
      | end
      | 
      | if strcmp(platformset(1),'_'),
      |     editvalStr = get_param(gcb,'editvalue_p');
      |     set_param(gcb,'platform_val',editvalStr);
      | else
      |     set_param(gcb,'platform_val',platformset);
      | end
      | 
      | if strcmp(categoryset(1),'_'),
      |     editvalStr = get_param(gcb,'editvalue_c');
      |     set_param(gcb,'algorithm_val',editvalStr);
      | else
      |     set_param(gcb,'algorithm_val',categoryset);
      | end
      mask Display:
      | val_dis_author = get_param(gcb,'author_val');
      | val_dis_plat = get_param(gcb,'platform_val');
      | val_dis_cat = get_param(gcb,'algorithm_val');
      | val_dis_desc = get_param(gcb,'AlgorithmFullName');
      | 
      | colorstr = 'black';
      | switch(val_dis_cat)
      |     case 'Management'
      |         colorstr = 'lightblue';
      |     case 'Prediction'
      |         colorstr = 'blue';
      |     case 'Control'
      |         colorstr = 'green';
      |     otherwise
      |         colorstr = 'yellow';
      | end
      | 
      | % if val_dis_cat == 'Management'
      | %     colorstr = 'lightblue';
      | % end
      | % if val_dis_cat == 'Prediction'
      | %     colorstr = 'blue';
      | % end
      | 
      | % if val_dis_cat == 'Control'
      | %     colorstr = 'blue';
      | % end
      | % if val_dis_cat == 'Control'
      | %     colorstr = 'green';
      | % end
      | 
      | color(colorstr);
      | text(0.5,0.9,val_dis_desc,'horizontalAlignment', 'center', 'VerticalAlignment','Top');
      | color('black');
      | fprintf('\nAuthor: %s\nPlatform: %s\nCategory: %s',val_dis_author,val_dis_plat,val_dis_cat);
  "ITS_convergence " : Subsystem  mask{AlgorithmFullName=EgoVehicle, pop_author=__UserDef, editvalue_a=user_define_author, pop_platform=MATLAB, editvalue_p=user_define_platform, pop_category=Management, editvalue_c=user_define_category, author_val=user_define_author, platform_val=MATLAB, algorithm_val=Management}
      mask prompts: pop_author "Author"; editvalue_a "UserDefine"; pop_platform "Platform"; editvalue_p "UserDefine"; pop_category "Category"; editvalue_c "UserDefine"; author_val "Buff_author"; platform_val "Buff_Platform"; algorithm_val "Buff_Category"
      mask TypeOptions pop_author: Kyunghan | Haksu | Kyuhwan | Gyubin | Seungeon | __UserDef
      mask Callback pop_author:
      | % Get the mask parameter values. This is a cell
      | %   array of character vectors.
      | authorStr = get_param(gcb,'pop_author');
      | % The pop-up menu is the first mask parameter.
      | %   Check the value selected in the pop-up
      | if strcmp(authorStr(1),'_'),
      |     % Set the visibility of both parameters on when
      |     %   User-defined is selected in the pop-up.
      |     set_param(gcb,'editvalue_a','user_define_author');
      |     set_param(gcb,'MaskVisibilities',{'on';'on';'on';'on';'off';'on';'off';'off';'off';'off'}),
      |     % Get all Tab Names returned in cell array
      | 
      |     % Get visibility of all parameters
      | %     editvalStr = get_param(gcb,'editvalue')
      | %     set_param(gcb,'author_val',editvalStr)
      | else
      | 
      |     % Turn off the visibility of the Value field
      |     %   when User-defined is not selected.
      | 
      |     set_param(gcb,'MaskVisibilities',{'on';'on';'off';'on';'off';'on';'off';'off';'off';'off'}),
      |     % Set the character vector in the Values field equal to the
      |     % character vector selected in the Gain pop-up menu.
      | 
      |     %maskStr{2}=maskStr{1};
      | %     set_param(gcb,'author_val',authorStr);
      | end
      mask TypeOptions pop_platform: MATLAB | Python | Visual_C | __UserDef
      mask Callback pop_platform:
      | % Get the mask parameter values. This is a cell
      | %   array of character vectors.
      | platformSet = get_param(gcb,'pop_platform');
      | % The pop-up menu is the first mask parameter.
      | %   Check the value selected in the pop-up
      | if strcmp(platformSet(1),'_'),
      |     % Set the visibility of both parameters on when
      |     %   User-defined is selected in the pop-up.
      |     set_param(gcb,'editvalue_p','user_define_platform')
      |     set_param(gcb,'MaskVisibilities',{'on';'on';'off';'on';'on';'on';'off';'off';'off';'off'}),
      |     % Get all Tab Names returned in cell array
      | 
      |     % Get visibility of all parameters
      | %     editvalStr = get_param(gcb,'editvalue')
      | %     set_param(gcb,'platform_val',editvalStr)
      | else
      | 
      |     % Turn off the visibility of the Value field
      |     %   when User-defined is not selected.
      | 
      |     set_param(gcb,'MaskVisibilities',{'on';'on';'off';'on';'off';'on';'off';'off';'off';'off'}),
      |     % Set the character vector in the Values field equal to the
      |     % character vector selected in the Gain pop-up menu.
      | 
      |     %maskStr{2}=maskStr{1};
      | %     set_param(gcb,'platform_val',platformSet);
      | end
      mask TypeOptions pop_category: Management | Prediction | Control | __UserDef
      mask Callback pop_category:
      | % Get the mask parameter values. This is a cell
      | %   array of character vectors.
      | categoryset = get_param(gcb,'pop_category');
      | % The pop-up menu is the first mask parameter.
      | %   Check the value selected in the pop-up
      | if strcmp(categoryset(1),'_'),
      |     % Set the visibility of both parameters on when
      |     %   User-defined is selected in the pop-up.
      |     set_param(gcb,'editvalue_c','user_define_category')
      |     set_param(gcb,'MaskVisibilities',{'on';'on';'off';'on';'off';'on';'on';'off';'off';'off'}),
      |     % Get all Tab Names returned in cell array
      | else
      |     % Turn off the visibility of the Value field
      |     %   when User-defined is not selected.
      |     set_param(gcb,'MaskVisibilities',{'on';'on';'off';'on';'off';'on';'off';'off';'off';'off'}),
      |     % Set the character vector in the Values field equal to the
      |     % character vector selected in the Gain pop-up menu.
      |     %maskStr{2}=maskStr{1};
      | end
      mask DialogControl DescGroupVar Prompt: Description
      mask DialogControl DescTextVar Prompt: %<AlgorithmFullName>
      mask DialogControl ParamDesc Prompt: Description
      mask DialogControl Text1 Prompt: Author: %<author_val>
      mask DialogControl Text2 Prompt: Platform: %<platform_val>
      mask DialogControl Text3 Prompt: Algorithm: %<algorithm_val>
      mask DialogControl ParameterGroupVar Prompt: SetParam
      mask DialogControl Control5 Prompt: Set
      mask DialogControl Control5 Callback:
      | authorset = get_param(gcb,'pop_author');
      | platformset = get_param(gcb,'pop_platform');
      | categoryset = get_param(gcb,'pop_category');
      | % The pop-up menu is the first mask parameter.
      | %   Check the value selected in the pop-up
      | if strcmp(authorset(1),'_'),
      |     editvalStr = get_param(gcb,'editvalue_a');
      |     set_param(gcb,'author_val',editvalStr);
      | else
      |     set_param(gcb,'author_val',authorset);
      | end
      | 
      | if strcmp(platformset(1),'_'),
      |     editvalStr = get_param(gcb,'editvalue_p');
      |     set_param(gcb,'platform_val',editvalStr);
      | else
      |     set_param(gcb,'platform_val',platformset);
      | end
      | 
      | if strcmp(categoryset(1),'_'),
      |     editvalStr = get_param(gcb,'editvalue_c');
      |     set_param(gcb,'algorithm_val',editvalStr);
      | else
      |     set_param(gcb,'algorithm_val',categoryset);
      | end
      mask Display:
      | val_dis_author = get_param(gcb,'author_val');
      | val_dis_plat = get_param(gcb,'platform_val');
      | val_dis_cat = get_param(gcb,'algorithm_val');
      | val_dis_desc = get_param(gcb,'AlgorithmFullName');
      | 
      | colorstr = 'black';
      | switch(val_dis_cat)
      |     case 'Management'
      |         colorstr = 'lightblue';
      |     case 'Prediction'
      |         colorstr = 'blue';
      |     case 'Control'
      |         colorstr = 'green';
      |     otherwise
      |         colorstr = 'yellow';
      | end
      | 
      | % if val_dis_cat == 'Management'
      | %     colorstr = 'lightblue';
      | % end
      | % if val_dis_cat == 'Prediction'
      | %     colorstr = 'blue';
      | % end
      | 
      | % if val_dis_cat == 'Control'
      | %     colorstr = 'blue';
      | % end
      | % if val_dis_cat == 'Control'
      | %     colorstr = 'green';
      | % end
      | 
      | color(colorstr);
      | text(0.5,0.9,val_dis_desc,'horizontalAlignment', 'center', 'VerticalAlignment','Top');
      | color('black');
      | fprintf('\nAuthor: %s\nPlatform: %s\nCategory: %s',val_dis_author,val_dis_plat,val_dis_cat);
  ITS_convergence 1 : Subsystem  mask{AlgorithmFullName=PrecedingVehicle, pop_author=__UserDef, editvalue_a=user_define_author, pop_platform=MATLAB, editvalue_p=user_define_platform, pop_category=Management, editvalue_c=user_define_category, author_val=user_define_author, platform_val=MATLAB, algorithm_val=Management}
      mask prompts: pop_author "Author"; editvalue_a "UserDefine"; pop_platform "Platform"; editvalue_p "UserDefine"; pop_category "Category"; editvalue_c "UserDefine"; author_val "Buff_author"; platform_val "Buff_Platform"; algorithm_val "Buff_Category"
      mask TypeOptions pop_author: Kyunghan | Haksu | Kyuhwan | Gyubin | Seungeon | __UserDef
      mask Callback pop_author:
      | % Get the mask parameter values. This is a cell
      | %   array of character vectors.
      | authorStr = get_param(gcb,'pop_author');
      | % The pop-up menu is the first mask parameter.
      | %   Check the value selected in the pop-up
      | if strcmp(authorStr(1),'_'),
      |     % Set the visibility of both parameters on when
      |     %   User-defined is selected in the pop-up.
      |     set_param(gcb,'editvalue_a','user_define_author');
      |     set_param(gcb,'MaskVisibilities',{'on';'on';'on';'on';'off';'on';'off';'off';'off';'off'}),
      |     % Get all Tab Names returned in cell array
      | 
      |     % Get visibility of all parameters
      | %     editvalStr = get_param(gcb,'editvalue')
      | %     set_param(gcb,'author_val',editvalStr)
      | else
      | 
      |     % Turn off the visibility of the Value field
      |     %   when User-defined is not selected.
      | 
      |     set_param(gcb,'MaskVisibilities',{'on';'on';'off';'on';'off';'on';'off';'off';'off';'off'}),
      |     % Set the character vector in the Values field equal to the
      |     % character vector selected in the Gain pop-up menu.
      | 
      |     %maskStr{2}=maskStr{1};
      | %     set_param(gcb,'author_val',authorStr);
      | end
      mask TypeOptions pop_platform: MATLAB | Python | Visual_C | __UserDef
      mask Callback pop_platform:
      | % Get the mask parameter values. This is a cell
      | %   array of character vectors.
      | platformSet = get_param(gcb,'pop_platform');
      | % The pop-up menu is the first mask parameter.
      | %   Check the value selected in the pop-up
      | if strcmp(platformSet(1),'_'),
      |     % Set the visibility of both parameters on when
      |     %   User-defined is selected in the pop-up.
      |     set_param(gcb,'editvalue_p','user_define_platform')
      |     set_param(gcb,'MaskVisibilities',{'on';'on';'off';'on';'on';'on';'off';'off';'off';'off'}),
      |     % Get all Tab Names returned in cell array
      | 
      |     % Get visibility of all parameters
      | %     editvalStr = get_param(gcb,'editvalue')
      | %     set_param(gcb,'platform_val',editvalStr)
      | else
      | 
      |     % Turn off the visibility of the Value field
      |     %   when User-defined is not selected.
      | 
      |     set_param(gcb,'MaskVisibilities',{'on';'on';'off';'on';'off';'on';'off';'off';'off';'off'}),
      |     % Set the character vector in the Values field equal to the
      |     % character vector selected in the Gain pop-up menu.
      | 
      |     %maskStr{2}=maskStr{1};
      | %     set_param(gcb,'platform_val',platformSet);
      | end
      mask TypeOptions pop_category: Management | Prediction | Control | __UserDef
      mask Callback pop_category:
      | % Get the mask parameter values. This is a cell
      | %   array of character vectors.
      | categoryset = get_param(gcb,'pop_category');
      | % The pop-up menu is the first mask parameter.
      | %   Check the value selected in the pop-up
      | if strcmp(categoryset(1),'_'),
      |     % Set the visibility of both parameters on when
      |     %   User-defined is selected in the pop-up.
      |     set_param(gcb,'editvalue_c','user_define_category')
      |     set_param(gcb,'MaskVisibilities',{'on';'on';'off';'on';'off';'on';'on';'off';'off';'off'}),
      |     % Get all Tab Names returned in cell array
      | else
      |     % Turn off the visibility of the Value field
      |     %   when User-defined is not selected.
      |     set_param(gcb,'MaskVisibilities',{'on';'on';'off';'on';'off';'on';'off';'off';'off';'off'}),
      |     % Set the character vector in the Values field equal to the
      |     % character vector selected in the Gain pop-up menu.
      |     %maskStr{2}=maskStr{1};
      | end
      mask DialogControl DescGroupVar Prompt: Description
      mask DialogControl DescTextVar Prompt: %<AlgorithmFullName>
      mask DialogControl ParamDesc Prompt: Description
      mask DialogControl Text1 Prompt: Author: %<author_val>
      mask DialogControl Text2 Prompt: Platform: %<platform_val>
      mask DialogControl Text3 Prompt: Algorithm: %<algorithm_val>
      mask DialogControl ParameterGroupVar Prompt: SetParam
      mask DialogControl Control5 Prompt: Set
      mask DialogControl Control5 Callback:
      | authorset = get_param(gcb,'pop_author');
      | platformset = get_param(gcb,'pop_platform');
      | categoryset = get_param(gcb,'pop_category');
      | % The pop-up menu is the first mask parameter.
      | %   Check the value selected in the pop-up
      | if strcmp(authorset(1),'_'),
      |     editvalStr = get_param(gcb,'editvalue_a');
      |     set_param(gcb,'author_val',editvalStr);
      | else
      |     set_param(gcb,'author_val',authorset);
      | end
      | 
      | if strcmp(platformset(1),'_'),
      |     editvalStr = get_param(gcb,'editvalue_p');
      |     set_param(gcb,'platform_val',editvalStr);
      | else
      |     set_param(gcb,'platform_val',platformset);
      | end
      | 
      | if strcmp(categoryset(1),'_'),
      |     editvalStr = get_param(gcb,'editvalue_c');
      |     set_param(gcb,'algorithm_val',editvalStr);
      | else
      |     set_param(gcb,'algorithm_val',categoryset);
      | end
      mask Display:
      | val_dis_author = get_param(gcb,'author_val');
      | val_dis_plat = get_param(gcb,'platform_val');
      | val_dis_cat = get_param(gcb,'algorithm_val');
      | val_dis_desc = get_param(gcb,'AlgorithmFullName');
      | 
      | colorstr = 'black';
      | switch(val_dis_cat)
      |     case 'Management'
      |         colorstr = 'lightblue';
      |     case 'Prediction'
      |         colorstr = 'blue';
      |     case 'Control'
      |         colorstr = 'green';
      |     otherwise
      |         colorstr = 'yellow';
      | end
      | 
      | % if val_dis_cat == 'Management'
      | %     colorstr = 'lightblue';
      | % end
      | % if val_dis_cat == 'Prediction'
      | %     colorstr = 'blue';
      | % end
      | 
      | % if val_dis_cat == 'Control'
      | %     colorstr = 'blue';
      | % end
      | % if val_dis_cat == 'Control'
      | %     colorstr = 'green';
      | % end
      | 
      | color(colorstr);
      | text(0.5,0.9,val_dis_desc,'horizontalAlignment', 'center', 'VerticalAlignment','Top');
      | color('black');
      | fprintf('\nAuthor: %s\nPlatform: %s\nCategory: %s',val_dis_author,val_dis_plat,val_dis_cat);
  ITS_convergence 2 : Subsystem  mask{AlgorithmFullName=Obstacles, pop_author=__UserDef, editvalue_a=user_define_author, pop_platform=MATLAB, editvalue_p=user_define_platform, pop_category=Management, editvalue_c=user_define_category, author_val=user_define_author, platform_val=MATLAB, algorithm_val=Management}
      mask prompts: pop_author "Author"; editvalue_a "UserDefine"; pop_platform "Platform"; editvalue_p "UserDefine"; pop_category "Category"; editvalue_c "UserDefine"; author_val "Buff_author"; platform_val "Buff_Platform"; algorithm_val "Buff_Category"
      mask TypeOptions pop_author: Kyunghan | Haksu | Kyuhwan | Gyubin | Seungeon | __UserDef
      mask Callback pop_author:
      | % Get the mask parameter values. This is a cell
      | %   array of character vectors.
      | authorStr = get_param(gcb,'pop_author');
      | % The pop-up menu is the first mask parameter.
      | %   Check the value selected in the pop-up
      | if strcmp(authorStr(1),'_'),
      |     % Set the visibility of both parameters on when
      |     %   User-defined is selected in the pop-up.
      |     set_param(gcb,'editvalue_a','user_define_author');
      |     set_param(gcb,'MaskVisibilities',{'on';'on';'on';'on';'off';'on';'off';'off';'off';'off'}),
      |     % Get all Tab Names returned in cell array
      | 
      |     % Get visibility of all parameters
      | %     editvalStr = get_param(gcb,'editvalue')
      | %     set_param(gcb,'author_val',editvalStr)
      | else
      | 
      |     % Turn off the visibility of the Value field
      |     %   when User-defined is not selected.
      | 
      |     set_param(gcb,'MaskVisibilities',{'on';'on';'off';'on';'off';'on';'off';'off';'off';'off'}),
      |     % Set the character vector in the Values field equal to the
      |     % character vector selected in the Gain pop-up menu.
      | 
      |     %maskStr{2}=maskStr{1};
      | %     set_param(gcb,'author_val',authorStr);
      | end
      mask TypeOptions pop_platform: MATLAB | Python | Visual_C | __UserDef
      mask Callback pop_platform:
      | % Get the mask parameter values. This is a cell
      | %   array of character vectors.
      | platformSet = get_param(gcb,'pop_platform');
      | % The pop-up menu is the first mask parameter.
      | %   Check the value selected in the pop-up
      | if strcmp(platformSet(1),'_'),
      |     % Set the visibility of both parameters on when
      |     %   User-defined is selected in the pop-up.
      |     set_param(gcb,'editvalue_p','user_define_platform')
      |     set_param(gcb,'MaskVisibilities',{'on';'on';'off';'on';'on';'on';'off';'off';'off';'off'}),
      |     % Get all Tab Names returned in cell array
      | 
      |     % Get visibility of all parameters
      | %     editvalStr = get_param(gcb,'editvalue')
      | %     set_param(gcb,'platform_val',editvalStr)
      | else
      | 
      |     % Turn off the visibility of the Value field
      |     %   when User-defined is not selected.
      | 
      |     set_param(gcb,'MaskVisibilities',{'on';'on';'off';'on';'off';'on';'off';'off';'off';'off'}),
      |     % Set the character vector in the Values field equal to the
      |     % character vector selected in the Gain pop-up menu.
      | 
      |     %maskStr{2}=maskStr{1};
      | %     set_param(gcb,'platform_val',platformSet);
      | end
      mask TypeOptions pop_category: Management | Prediction | Control | __UserDef
      mask Callback pop_category:
      | % Get the mask parameter values. This is a cell
      | %   array of character vectors.
      | categoryset = get_param(gcb,'pop_category');
      | % The pop-up menu is the first mask parameter.
      | %   Check the value selected in the pop-up
      | if strcmp(categoryset(1),'_'),
      |     % Set the visibility of both parameters on when
      |     %   User-defined is selected in the pop-up.
      |     set_param(gcb,'editvalue_c','user_define_category')
      |     set_param(gcb,'MaskVisibilities',{'on';'on';'off';'on';'off';'on';'on';'off';'off';'off'}),
      |     % Get all Tab Names returned in cell array
      | else
      |     % Turn off the visibility of the Value field
      |     %   when User-defined is not selected.
      |     set_param(gcb,'MaskVisibilities',{'on';'on';'off';'on';'off';'on';'off';'off';'off';'off'}),
      |     % Set the character vector in the Values field equal to the
      |     % character vector selected in the Gain pop-up menu.
      |     %maskStr{2}=maskStr{1};
      | end
      mask DialogControl DescGroupVar Prompt: Description
      mask DialogControl DescTextVar Prompt: %<AlgorithmFullName>
      mask DialogControl ParamDesc Prompt: Description
      mask DialogControl Text1 Prompt: Author: %<author_val>
      mask DialogControl Text2 Prompt: Platform: %<platform_val>
      mask DialogControl Text3 Prompt: Algorithm: %<algorithm_val>
      mask DialogControl ParameterGroupVar Prompt: SetParam
      mask DialogControl Control5 Prompt: Set
      mask DialogControl Control5 Callback:
      | authorset = get_param(gcb,'pop_author');
      | platformset = get_param(gcb,'pop_platform');
      | categoryset = get_param(gcb,'pop_category');
      | % The pop-up menu is the first mask parameter.
      | %   Check the value selected in the pop-up
      | if strcmp(authorset(1),'_'),
      |     editvalStr = get_param(gcb,'editvalue_a');
      |     set_param(gcb,'author_val',editvalStr);
      | else
      |     set_param(gcb,'author_val',authorset);
      | end
      | 
      | if strcmp(platformset(1),'_'),
      |     editvalStr = get_param(gcb,'editvalue_p');
      |     set_param(gcb,'platform_val',editvalStr);
      | else
      |     set_param(gcb,'platform_val',platformset);
      | end
      | 
      | if strcmp(categoryset(1),'_'),
      |     editvalStr = get_param(gcb,'editvalue_c');
      |     set_param(gcb,'algorithm_val',editvalStr);
      | else
      |     set_param(gcb,'algorithm_val',categoryset);
      | end
      mask Display:
      | val_dis_author = get_param(gcb,'author_val');
      | val_dis_plat = get_param(gcb,'platform_val');
      | val_dis_cat = get_param(gcb,'algorithm_val');
      | val_dis_desc = get_param(gcb,'AlgorithmFullName');
      | 
      | colorstr = 'black';
      | switch(val_dis_cat)
      |     case 'Management'
      |         colorstr = 'lightblue';
      |     case 'Prediction'
      |         colorstr = 'blue';
      |     case 'Control'
      |         colorstr = 'green';
      |     otherwise
      |         colorstr = 'yellow';
      | end
      | 
      | % if val_dis_cat == 'Management'
      | %     colorstr = 'lightblue';
      | % end
      | % if val_dis_cat == 'Prediction'
      | %     colorstr = 'blue';
      | % end
      | 
      | % if val_dis_cat == 'Control'
      | %     colorstr = 'blue';
      | % end
      | % if val_dis_cat == 'Control'
      | %     colorstr = 'green';
      | % end
      | 
      | color(colorstr);
      | text(0.5,0.9,val_dis_desc,'horizontalAlignment', 'center', 'VerticalAlignment','Top');
      | color('black');
      | fprintf('\nAuthor: %s\nPlatform: %s\nCategory: %s',val_dis_author,val_dis_plat,val_dis_cat);
  ITS_convergence 3 : Subsystem  mask{AlgorithmFullName=Topography, pop_author=__UserDef, editvalue_a=user_define_author, pop_platform=MATLAB, editvalue_p=user_define_platform, pop_category=Management, editvalue_c=user_define_category, author_val=user_define_author, platform_val=MATLAB, algorithm_val=Management}
      mask prompts: pop_author "Author"; editvalue_a "UserDefine"; pop_platform "Platform"; editvalue_p "UserDefine"; pop_category "Category"; editvalue_c "UserDefine"; author_val "Buff_author"; platform_val "Buff_Platform"; algorithm_val "Buff_Category"
      mask TypeOptions pop_author: Kyunghan | Haksu | Kyuhwan | Gyubin | Seungeon | __UserDef
      mask Callback pop_author:
      | % Get the mask parameter values. This is a cell
      | %   array of character vectors.
      | authorStr = get_param(gcb,'pop_author');
      | % The pop-up menu is the first mask parameter.
      | %   Check the value selected in the pop-up
      | if strcmp(authorStr(1),'_'),
      |     % Set the visibility of both parameters on when
      |     %   User-defined is selected in the pop-up.
      |     set_param(gcb,'editvalue_a','user_define_author');
      |     set_param(gcb,'MaskVisibilities',{'on';'on';'on';'on';'off';'on';'off';'off';'off';'off'}),
      |     % Get all Tab Names returned in cell array
      | 
      |     % Get visibility of all parameters
      | %     editvalStr = get_param(gcb,'editvalue')
      | %     set_param(gcb,'author_val',editvalStr)
      | else
      | 
      |     % Turn off the visibility of the Value field
      |     %   when User-defined is not selected.
      | 
      |     set_param(gcb,'MaskVisibilities',{'on';'on';'off';'on';'off';'on';'off';'off';'off';'off'}),
      |     % Set the character vector in the Values field equal to the
      |     % character vector selected in the Gain pop-up menu.
      | 
      |     %maskStr{2}=maskStr{1};
      | %     set_param(gcb,'author_val',authorStr);
      | end
      mask TypeOptions pop_platform: MATLAB | Python | Visual_C | __UserDef
      mask Callback pop_platform:
      | % Get the mask parameter values. This is a cell
      | %   array of character vectors.
      | platformSet = get_param(gcb,'pop_platform');
      | % The pop-up menu is the first mask parameter.
      | %   Check the value selected in the pop-up
      | if strcmp(platformSet(1),'_'),
      |     % Set the visibility of both parameters on when
      |     %   User-defined is selected in the pop-up.
      |     set_param(gcb,'editvalue_p','user_define_platform')
      |     set_param(gcb,'MaskVisibilities',{'on';'on';'off';'on';'on';'on';'off';'off';'off';'off'}),
      |     % Get all Tab Names returned in cell array
      | 
      |     % Get visibility of all parameters
      | %     editvalStr = get_param(gcb,'editvalue')
      | %     set_param(gcb,'platform_val',editvalStr)
      | else
      | 
      |     % Turn off the visibility of the Value field
      |     %   when User-defined is not selected.
      | 
      |     set_param(gcb,'MaskVisibilities',{'on';'on';'off';'on';'off';'on';'off';'off';'off';'off'}),
      |     % Set the character vector in the Values field equal to the
      |     % character vector selected in the Gain pop-up menu.
      | 
      |     %maskStr{2}=maskStr{1};
      | %     set_param(gcb,'platform_val',platformSet);
      | end
      mask TypeOptions pop_category: Management | Prediction | Control | __UserDef
      mask Callback pop_category:
      | % Get the mask parameter values. This is a cell
      | %   array of character vectors.
      | categoryset = get_param(gcb,'pop_category');
      | % The pop-up menu is the first mask parameter.
      | %   Check the value selected in the pop-up
      | if strcmp(categoryset(1),'_'),
      |     % Set the visibility of both parameters on when
      |     %   User-defined is selected in the pop-up.
      |     set_param(gcb,'editvalue_c','user_define_category')
      |     set_param(gcb,'MaskVisibilities',{'on';'on';'off';'on';'off';'on';'on';'off';'off';'off'}),
      |     % Get all Tab Names returned in cell array
      | else
      |     % Turn off the visibility of the Value field
      |     %   when User-defined is not selected.
      |     set_param(gcb,'MaskVisibilities',{'on';'on';'off';'on';'off';'on';'off';'off';'off';'off'}),
      |     % Set the character vector in the Values field equal to the
      |     % character vector selected in the Gain pop-up menu.
      |     %maskStr{2}=maskStr{1};
      | end
      mask DialogControl DescGroupVar Prompt: Description
      mask DialogControl DescTextVar Prompt: %<AlgorithmFullName>
      mask DialogControl ParamDesc Prompt: Description
      mask DialogControl Text1 Prompt: Author: %<author_val>
      mask DialogControl Text2 Prompt: Platform: %<platform_val>
      mask DialogControl Text3 Prompt: Algorithm: %<algorithm_val>
      mask DialogControl ParameterGroupVar Prompt: SetParam
      mask DialogControl Control5 Prompt: Set
      mask DialogControl Control5 Callback:
      | authorset = get_param(gcb,'pop_author');
      | platformset = get_param(gcb,'pop_platform');
      | categoryset = get_param(gcb,'pop_category');
      | % The pop-up menu is the first mask parameter.
      | %   Check the value selected in the pop-up
      | if strcmp(authorset(1),'_'),
      |     editvalStr = get_param(gcb,'editvalue_a');
      |     set_param(gcb,'author_val',editvalStr);
      | else
      |     set_param(gcb,'author_val',authorset);
      | end
      | 
      | if strcmp(platformset(1),'_'),
      |     editvalStr = get_param(gcb,'editvalue_p');
      |     set_param(gcb,'platform_val',editvalStr);
      | else
      |     set_param(gcb,'platform_val',platformset);
      | end
      | 
      | if strcmp(categoryset(1),'_'),
      |     editvalStr = get_param(gcb,'editvalue_c');
      |     set_param(gcb,'algorithm_val',editvalStr);
      | else
      |     set_param(gcb,'algorithm_val',categoryset);
      | end
      mask Display:
      | val_dis_author = get_param(gcb,'author_val');
      | val_dis_plat = get_param(gcb,'platform_val');
      | val_dis_cat = get_param(gcb,'algorithm_val');
      | val_dis_desc = get_param(gcb,'AlgorithmFullName');
      | 
      | colorstr = 'black';
      | switch(val_dis_cat)
      |     case 'Management'
      |         colorstr = 'lightblue';
      |     case 'Prediction'
      |         colorstr = 'blue';
      |     case 'Control'
      |         colorstr = 'green';
      |     otherwise
      |         colorstr = 'yellow';
      | end
      | 
      | % if val_dis_cat == 'Management'
      | %     colorstr = 'lightblue';
      | % end
      | % if val_dis_cat == 'Prediction'
      | %     colorstr = 'blue';
      | % end
      | 
      | % if val_dis_cat == 'Control'
      | %     colorstr = 'blue';
      | % end
      | % if val_dis_cat == 'Control'
      | %     colorstr = 'green';
      | % end
      | 
      | color(colorstr);
      | text(0.5,0.9,val_dis_desc,'horizontalAlignment', 'center', 'VerticalAlignment','Top');
      | color('black');
      | fprintf('\nAuthor: %s\nPlatform: %s\nCategory: %s',val_dis_author,val_dis_plat,val_dis_cat);
  Model Info : DX_Lib/Misc. Lib/Model Info  InitialBlockCM=None  BlockCM=None  Frame=on  DisplayStringWithTags=|  HorizontalTextAlignment=Left  LeftAlignmentValue=0.02  SourceBlockDiagram=DX_Lib  TagMaxNumber=20
      | * Model description: %<Description>
      |   1. Design. : x.doc, Ver x.x
      |   2. Created %<Created> by %<Creator>
      |   3. Modfied %<ModifiedDate> by %<ModifiedBy>
      |   4. Model version:  Ver. %<ModelVersion>
      settings: SourceProductName=ACE Lab: DX Blockset
  Mux : Mux  Inputs=2
  Mux1 : Mux  Inputs=2
  Mux2 : Mux
  Mux3 : Mux  Inputs=3
  "Static State " : Subsystem  mask{AlgorithmFullName=EgoVeh_State, pop_author=__UserDef, editvalue_a=user_define_author, pop_platform=Python, editvalue_p=user_define_platform, pop_category=Management, editvalue_c=user_define_category, author_val=user_define_author, platform_val=Python, algorithm_val=Management}
      mask prompts: pop_author "Author"; editvalue_a "UserDefine"; pop_platform "Platform"; editvalue_p "UserDefine"; pop_category "Category"; editvalue_c "UserDefine"; author_val "Buff_author"; platform_val "Buff_Platform"; algorithm_val "Buff_Category"
      mask TypeOptions pop_author: Kyunghan | Haksu | Kyuhwan | Gyubin | Seungeon | __UserDef
      mask Callback pop_author:
      | % Get the mask parameter values. This is a cell
      | %   array of character vectors.
      | authorStr = get_param(gcb,'pop_author');
      | % The pop-up menu is the first mask parameter.
      | %   Check the value selected in the pop-up
      | if strcmp(authorStr(1),'_'),
      |     % Set the visibility of both parameters on when
      |     %   User-defined is selected in the pop-up.
      |     set_param(gcb,'editvalue_a','user_define_author');
      |     set_param(gcb,'MaskVisibilities',{'on';'on';'on';'on';'off';'on';'off';'off';'off';'off'}),
      |     % Get all Tab Names returned in cell array
      | 
      |     % Get visibility of all parameters
      | %     editvalStr = get_param(gcb,'editvalue')
      | %     set_param(gcb,'author_val',editvalStr)
      | else
      | 
      |     % Turn off the visibility of the Value field
      |     %   when User-defined is not selected.
      | 
      |     set_param(gcb,'MaskVisibilities',{'on';'on';'off';'on';'off';'on';'off';'off';'off';'off'}),
      |     % Set the character vector in the Values field equal to the
      |     % character vector selected in the Gain pop-up menu.
      | 
      |     %maskStr{2}=maskStr{1};
      | %     set_param(gcb,'author_val',authorStr);
      | end
      mask TypeOptions pop_platform: MATLAB | Python | Visual_C | __UserDef
      mask Callback pop_platform:
      | % Get the mask parameter values. This is a cell
      | %   array of character vectors.
      | platformSet = get_param(gcb,'pop_platform');
      | % The pop-up menu is the first mask parameter.
      | %   Check the value selected in the pop-up
      | if strcmp(platformSet(1),'_'),
      |     % Set the visibility of both parameters on when
      |     %   User-defined is selected in the pop-up.
      |     set_param(gcb,'editvalue_p','user_define_platform')
      |     set_param(gcb,'MaskVisibilities',{'on';'on';'off';'on';'on';'on';'off';'off';'off';'off'}),
      |     % Get all Tab Names returned in cell array
      | 
      |     % Get visibility of all parameters
      | %     editvalStr = get_param(gcb,'editvalue')
      | %     set_param(gcb,'platform_val',editvalStr)
      | else
      | 
      |     % Turn off the visibility of the Value field
      |     %   when User-defined is not selected.
      | 
      |     set_param(gcb,'MaskVisibilities',{'on';'on';'off';'on';'off';'on';'off';'off';'off';'off'}),
      |     % Set the character vector in the Values field equal to the
      |     % character vector selected in the Gain pop-up menu.
      | 
      |     %maskStr{2}=maskStr{1};
      | %     set_param(gcb,'platform_val',platformSet);
      | end
      mask TypeOptions pop_category: Management | Prediction | Control | __UserDef
      mask Callback pop_category:
      | % Get the mask parameter values. This is a cell
      | %   array of character vectors.
      | categoryset = get_param(gcb,'pop_category');
      | % The pop-up menu is the first mask parameter.
      | %   Check the value selected in the pop-up
      | if strcmp(categoryset(1),'_'),
      |     % Set the visibility of both parameters on when
      |     %   User-defined is selected in the pop-up.
      |     set_param(gcb,'editvalue_c','user_define_category')
      |     set_param(gcb,'MaskVisibilities',{'on';'on';'off';'on';'off';'on';'on';'off';'off';'off'}),
      |     % Get all Tab Names returned in cell array
      | else
      |     % Turn off the visibility of the Value field
      |     %   when User-defined is not selected.
      |     set_param(gcb,'MaskVisibilities',{'on';'on';'off';'on';'off';'on';'off';'off';'off';'off'}),
      |     % Set the character vector in the Values field equal to the
      |     % character vector selected in the Gain pop-up menu.
      |     %maskStr{2}=maskStr{1};
      | end
      mask DialogControl DescGroupVar Prompt: Description
      mask DialogControl DescTextVar Prompt: %<AlgorithmFullName>
      mask DialogControl ParamDesc Prompt: Description
      mask DialogControl Text1 Prompt: Author: %<author_val>
      mask DialogControl Text2 Prompt: Platform: %<platform_val>
      mask DialogControl Text3 Prompt: Algorithm: %<algorithm_val>
      mask DialogControl ParameterGroupVar Prompt: SetParam
      mask DialogControl Control5 Prompt: Set
      mask DialogControl Control5 Callback:
      | authorset = get_param(gcb,'pop_author');
      | platformset = get_param(gcb,'pop_platform');
      | categoryset = get_param(gcb,'pop_category');
      | % The pop-up menu is the first mask parameter.
      | %   Check the value selected in the pop-up
      | if strcmp(authorset(1),'_'),
      |     editvalStr = get_param(gcb,'editvalue_a');
      |     set_param(gcb,'author_val',editvalStr);
      | else
      |     set_param(gcb,'author_val',authorset);
      | end
      | 
      | if strcmp(platformset(1),'_'),
      |     editvalStr = get_param(gcb,'editvalue_p');
      |     set_param(gcb,'platform_val',editvalStr);
      | else
      |     set_param(gcb,'platform_val',platformset);
      | end
      | 
      | if strcmp(categoryset(1),'_'),
      |     editvalStr = get_param(gcb,'editvalue_c');
      |     set_param(gcb,'algorithm_val',editvalStr);
      | else
      |     set_param(gcb,'algorithm_val',categoryset);
      | end
      mask Display:
      | val_dis_author = get_param(gcb,'author_val');
      | val_dis_plat = get_param(gcb,'platform_val');
      | val_dis_cat = get_param(gcb,'algorithm_val');
      | val_dis_desc = get_param(gcb,'AlgorithmFullName');
      | 
      | colorstr = 'black';
      | switch(val_dis_cat)
      |     case 'Management'
      |         colorstr = 'lightblue';
      |     case 'Prediction'
      |         colorstr = 'blue';
      |     case 'Control'
      |         colorstr = 'green';
      |     otherwise
      |         colorstr = 'yellow';
      | end
      | 
      | % if val_dis_cat == 'Management'
      | %     colorstr = 'lightblue';
      | % end
      | % if val_dis_cat == 'Prediction'
      | %     colorstr = 'blue';
      | % end
      | 
      | % if val_dis_cat == 'Control'
      | %     colorstr = 'blue';
      | % end
      | % if val_dis_cat == 'Control'
      | %     colorstr = 'green';
      | % end
      | 
      | color(colorstr);
      | text(0.5,0.9,val_dis_desc,'horizontalAlignment', 'center', 'VerticalAlignment','Top');
      | color('black');
      | fprintf('\nAuthor: %s\nPlatform: %s\nCategory: %s',val_dis_author,val_dis_plat,val_dis_cat);
  wires:
  Mux/1 -> ITS_convergence 3/1(In1), ITS_convergence 2/1(In1), ITS_convergence 1/1(In1), "ITS_convergence "/1(In1)
  <ArchitectureBlock>/1(Out1) -> Mux/1
  <ArchitectureBlock>2/1(Out1) -> Mux/2
  Mux1/1 -> <ArchitectureBlock>4/1(In1), <ArchitectureBlock>3/1(In1)
  "ITS_convergence "/1(Out1) -> Mux2/1
  ITS_convergence 1/1(Out1) -> Mux2/2
  ITS_convergence 2/1(Out1) -> Mux2/3
  ITS_convergence 3/1(Out1) -> Mux2/4
  Mux2/1 -> <ArchitectureBlock>5/1(In1), <ArchitectureBlock>1/1(In1), "Static State "/1(In1), Mux1/1
  <ArchitectureBlock>1/1(Out1) -> Mux3/2
  <ArchitectureBlock>5/1(Out1) -> Mux3/3
  "Static State "/1(Out1) -> Mux3/1
  Mux3/1 -> Mux1/2
